simulink model "ReynoldsNumber_TestModel"  (R2014a)
settings: Solver=ode45  StartTime=0.0  StopTime=10.0  RelTol=1e-3
libraries: rocket_drag_library x1
settings Model: Creator=scorpii  LastModifiedBy=scorpii

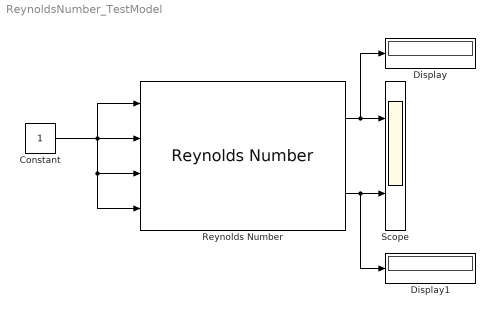
== system ReynoldsNumber_TestModel ==
  Constant : Constant
  Display : Display
  Display1 : Display
  Reynolds Number : rocket_drag_library/Reynolds Number
  Scope : Scope  NumInputPorts=2
      settings: YMin=-5~-5  YMax=5~5
  wires:
  Reynolds Number/1 -> Display/1, Scope/1
  Reynolds Number/2 -> Display1/1, Scope/2
  Constant/1 -> Reynolds Number/4, Reynolds Number/3, Reynolds Number/2, Reynolds Number/1
